simulink model "CanBusRagnarObserverPacketLoss"  (R2021b)
settings: Solver=VariableStepAuto  StartTime=0.0  StopTime=1.5  RelTol=1e-3
values from neighbouring files (symbols this model uses):
  F_mimo = -place(A,B,Desired_poles)    [SS_MIMO.m]
  L_mimo = -place(A',C',Desired_poles_obs)'    [SS_MIMO.m]
  sys_mimo = ss(A,B,C,0)    [SS_MIMO.m]
libraries: simulink_extras x8, truetime x6, dspsrcs4 x1
settings Model: Creator=mozzr  LastModifiedBy=mozzr
settings SolverCC: AlgebraicLoopSolver=TrustRegion

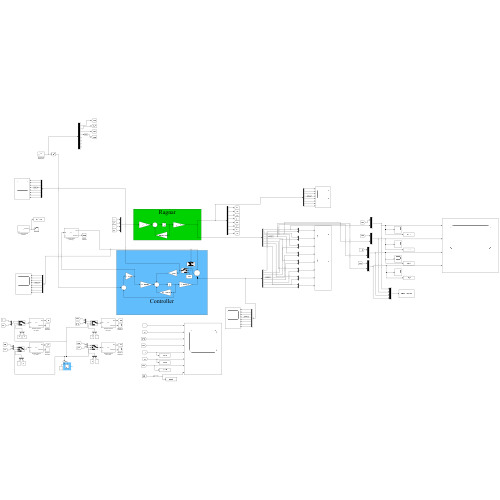
[thumbnail: Simulink's stored preview of the top-level diagram]
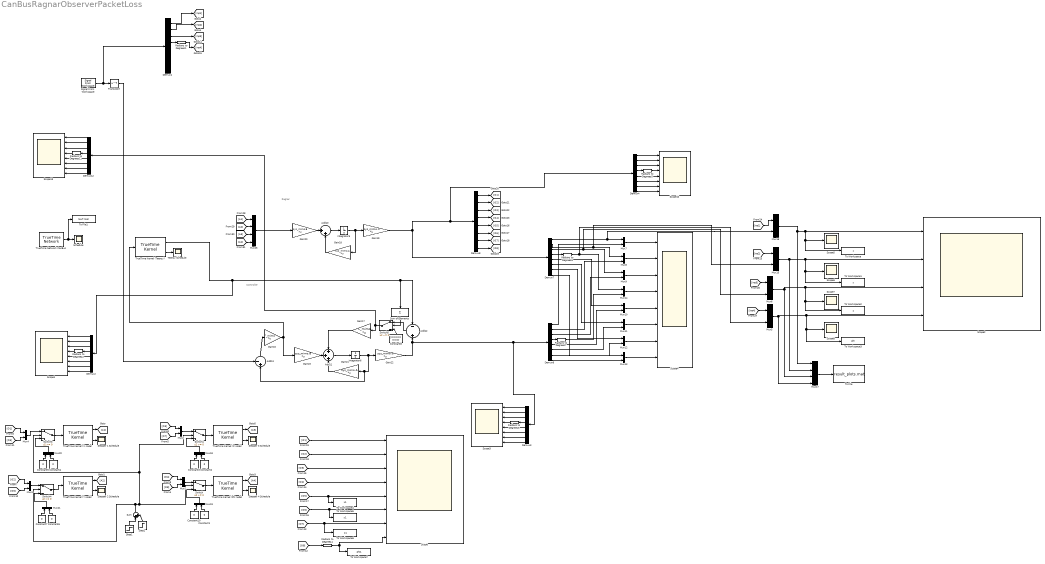
== system CanBusRagnarObserverPacketLoss ==
  note: Ragnar
  note: Controller
  Add10 : Sum  Inputs=|++
  Add11 : Sum  Inputs=+++
  Add12 : Sum  Inputs=-+
  Add13 : Sum  Inputs=-+|
  Constant{1..7,10} (8 alike) : Constant  Value=0
  Constant8 : Constant  Value=[0 0 0 0 0 0 0 0]'
  Demux{1..4,6..8,12} (8 alike) : Demux  Outputs=8
  Gain16 : Gain  Gain=F_mimo  Multiplication=Matrix(K*u)
  Gain17 : Gain  Gain=L_mimo  Multiplication=Matrix(K*u)
  Gain18 : Gain  Gain=sys_mimo.A  Multiplication=Matrix(K*u)
  Gain19 : Gain  Gain=sys_mimo.C  Multiplication=Matrix(K*u)
  Gain20 : Gain  Gain=sys_mimo.B  Multiplication=Matrix(K*u)
  Gain21 : Gain  Gain=sys_mimo.A  Multiplication=Matrix(K*u)
  Gain22 : Gain  Gain=sys_mimo.C  Multiplication=Matrix(K*u)
  Gain23 : Gain  Gain=sys_mimo.B  Multiplication=Matrix(K*u)
  Integrator5 : Integrator  InitialCondition=[0.01 0.51 -0.39 deg2rad(95) 0 0 0 0]'
  Integrator6 : Integrator  InitialCondition=[0.01 0.51 -0.39 deg2rad(95) 0 0 0 0]'
  Mux{1..16,18..21} (20 alike) : Mux  Inputs=2
  Mux17 : Mux
  Mux26 : Mux
  Radians to Degrees{1..7,11} (8 alike) : simulink_extras/Transformations/Radians to Degrees
  Schedule : Scope
  Scope{,1,3..4,10,13} (6 alike) : Scope  NumInputPorts=8
  Scope2 : Scope  NumInputPorts=4
  Scope{5..8} (4 alike) : Scope
  Signal From Workspace : dspsrcs4/Signal From Workspace  X=ref  Ts=0.5  nsamps=1  OutputAfterFinalValue=Holding final value  ignoreOrWarnInputAndFrameLengths=off  OutputFrames=off
  Step1 : Step  Time=0.7  Before=1  After=-1  SampleTime=0
  Step2 : Step  Time=0.9  After=2  SampleTime=0
  Stepper 1 Schedule : Scope
  Stepper 2 Schedule : Scope
  Stepper 3 Schedule : Scope
  Stepper 4 Schedule : Scope
  Sum : Sum  Inputs=|++
  Sum of Elements : Sum  Inputs=1
  Switch{,1,3..4} (4 alike) : Switch
  Switch5 : Switch  Criteria=u2 ~= 0  Threshold=1
  Teensy Schedule : Scope
  To File : ToFile  Filename=result_plots.mat  SaveFormat=Timeseries
  To File1 : ToFile  Filename=NwT.mat  SaveFormat=Timeseries
  To Workspace : ToWorkspace  VariableName=x  SaveFormat=Timeseries  SampleTime=-1
  To Workspace1 : ToWorkspace  VariableName=y  SaveFormat=Timeseries  SampleTime=-1
  To Workspace2 : ToWorkspace  VariableName=z  SaveFormat=Timeseries  SampleTime=-1
  To Workspace3 : ToWorkspace  VariableName=phi  SaveFormat=Timeseries  SampleTime=-1
  To Workspace4 : ToWorkspace  VariableName=x1  SaveFormat=Timeseries  SampleTime=-1
  To Workspace5 : ToWorkspace  VariableName=y1  SaveFormat=Timeseries  SampleTime=-1
  To Workspace6 : ToWorkspace  VariableName=z1  SaveFormat=Timeseries  SampleTime=-1
  To Workspace7 : ToWorkspace  VariableName=phi1  SaveFormat=Timeseries  SampleTime=-1
  Transpose : Math  Operator=transpose  SaturateOnIntegerOverflow=on
  TrueTime Kernel (Phi node) : truetime/TrueTime Kernel  sfun=nodePhi_init  args=[]  ninputsoutputs=[2 1]  ntriggers=0  trigtype=falling  nwnodenbr=[1 5]  clockoffsetdrift=[0 0]  schedoutput=on  battery=off  poweroutput=off  label=1: 5
  TrueTime Kernel (Teensy) : truetime/TrueTime Kernel  sfun=Teensy_init  args=[]  ninputsoutputs=[4 8]  ntriggers=0  trigtype=falling  nwnodenbr=[1 1]  clockoffsetdrift=[0 0]  schedoutput=on  battery=off  poweroutput=off  label=1: 1
  TrueTime Kernel (X node) : truetime/TrueTime Kernel  sfun=nodeX_init  args=[]  ninputsoutputs=[2 1]  ntriggers=0  trigtype=falling  nwnodenbr=[1 2]  clockoffsetdrift=[0 0]  schedoutput=on  battery=off  poweroutput=off  label=1: 2
  TrueTime Kernel (Y node) : truetime/TrueTime Kernel  sfun=nodeY_init  args=[]  ninputsoutputs=[2 1]  ntriggers=0  trigtype=falling  nwnodenbr=[1 3]  clockoffsetdrift=[0 0]  schedoutput=on  battery=off  poweroutput=off  label=1: 3
  TrueTime Kernel (Z node) : truetime/TrueTime Kernel  sfun=nodeZ_init  args=[]  ninputsoutputs=[2 1]  ntriggers=0  trigtype=falling  nwnodenbr=[1 4]  clockoffsetdrift=[0 0]  schedoutput=on  battery=off  poweroutput=off  label=1: 4
  TrueTime Network CanBus : truetime/TrueTime Network  nwtype=CSMA/AMP (CAN)  nwnbr=1  nnodes=5  rate=10000000  minsize=512  lossprob=0  seed=0  bandwidths=[0.5 0.5]  slotsize=512  schedule=[1 1 2]  memsize=80000  buftype=Common buffer  overflow=Retransmit  dynSchedule=0  miniSlotSize=0  NIT=0  QSortMode=FIFO  sync=0  irtSchedule=0  nrtLength=0  nodeGraph=0  scheduleoutput=on
  wires:
  TrueTime Kernel (Teensy)/2 -> Teensy Schedule/1
  TrueTime Network CanBus/1 -> To File1/1, Schedule/1
  [O7] -> To Workspace6/1, Scope/7
  [O4] -> Scope/4
  [O3] -> Scope/3
  [O5] -> To Workspace4/1, Scope/5
  [O6] -> To Workspace5/1, Scope/6
  [O2] -> Scope/2
  [O1] -> Scope/1
  Mux12/1 -> Scope4/7
  Mux7/1 -> Scope4/1
  Demux6/5 -> Mux10/2
  Mux11/1 -> Scope4/6
  Demux7/7 -> Mux12/1
  Demux6/1 -> Mux7/2
  Radians to Degrees7/1 -> Mux14/2
  Demux6/6 -> Mux11/2
  Demux6/7 -> Mux12/2
  Demux7/2 -> Mux15/2, Mux8/1
  Mux10/1 -> Scope4/5
  Demux6/2 -> Mux8/2
  Demux7/5 -> Mux10/1
  Mux13/1 -> Scope4/8
  Demux7/6 -> Mux11/1
  Radians to Degrees6/1 -> Mux5/2, Mux14/1
  Demux6/8 -> Mux13/2
  Demux7/8 -> Mux13/1
  Mux14/1 -> Scope4/4
  Demux6/4 -> Radians to Degrees7/1
  Demux6/3 -> Mux9/2
  Demux7/1 -> Mux16/2, Mux7/1
  Mux9/1 -> Scope4/3
  Demux7/4 -> Radians to Degrees6/1
  Demux7/3 -> Mux6/2, Mux9/1
  Mux8/1 -> Scope4/2
  Mux5/1 -> To Workspace3/1, Scope8/1, Scope2/4, Mux17/4
  Mux6/1 -> To Workspace2/1, Scope7/1, Scope2/3, Mux17/3
  Mux15/1 -> Mux17/2, To Workspace1/1, Scope6/1, Scope2/2
  Mux16/1 -> Mux17/1, To Workspace/1, Scope5/1, Scope2/1
  Demux1/4 -> Radians to Degrees1/1
  Demux1/1 -> [inp1]
  Demux1/2 -> [inp2]
  Demux1/3 -> [inp3]
  Radians to Degrees1/1 -> [inp4]
  [inp1] -> Mux16/1
  [inp2] -> Mux15/1
  [inp3] -> Mux6/1
  [inp4] -> Mux5/1
  Mux17/1 -> To File/1
  Gain21/1 -> Add11/3
  Add13/1 -> Gain16/1
  Gain23/1 -> Add11/2
  Gain16/1 -> TrueTime Kernel (Teensy)/1, Gain23/1
  Integrator5/1 -> Gain18/1, Gain19/1
  Gain18/1 -> Add10/2
  Gain20/1 -> Add10/1
  Add11/1 -> Integrator6/1
  Gain22/1 -> Demux3/1, Demux6/1, Add12/2
  Add10/1 -> Integrator5/1
  Gain17/1 -> Add11/1
  Integrator6/1 -> Add13/2, Gain21/1, Gain22/1
  Demux8/8 -> [O8]
  Demux8/7 -> [O7]
  Demux8/4 -> [O4]
  Demux8/5 -> [O5]
  Demux8/3 -> [O3]
  Demux8/1 -> [O1]
  Demux8/2 -> [O2]
  Demux8/6 -> [O6]
  [A4] -> Mux26/4
  [A3] -> Mux26/3
  [A2] -> Mux26/2
  [A1] -> Mux26/1
  Mux26/1 -> Gain20/1
  Signal From Workspace/1 -> Demux1/1, Transpose/1
  Transpose/1 -> Add13/1
  Demux4/6 -> Scope10/6
  Demux4/8 -> Scope10/8
  Demux4/2 -> Scope10/2
  Demux4/1 -> Scope10/1
  Demux4/7 -> Scope10/7
  Demux4/3 -> Scope10/3
  Demux4/4 -> Radians to Degrees5/1
  Demux4/5 -> Scope10/5
  Radians to Degrees5/1 -> Scope10/4
  Gain19/1 -> Demux4/1, Demux8/1, Demux7/1
  Demux12/6 -> Scope13/6
  Demux12/4 -> Radians to Degrees11/1
  Demux12/1 -> Scope13/1
  Demux12/8 -> Scope13/8
  Demux12/5 -> Scope13/5
  Radians to Degrees11/1 -> Scope13/4
  Demux12/2 -> Scope13/2
  Demux12/3 -> Scope13/3
  Demux12/7 -> Scope13/7
  [O2] -> Mux3/1
  Mux21/1 -> Switch4/3
  Constant7/1 -> Mux21/1
  [O1] -> Mux4/1
  Step1/1 -> Sum/1
  TrueTime Kernel (X node)/2 -> Stepper 1 Schedule/1
  Constant1/1 -> Mux19/2
  Constant5/1 -> Mux20/1
  Switch1/1 -> TrueTime Kernel (Z node)/1
  TrueTime Kernel (Phi node)/1 -> [A4]
  Mux20/1 -> Switch3/3
  Switch4/1 -> TrueTime Kernel (Y node)/1
  Constant4/1 -> Mux20/2
  Mux3/1 -> Switch4/1
  [O8] -> Mux1/2
  Mux4/1 -> Switch3/1
  Mux18/1 -> Switch1/3
  Constant2/1 -> Mux18/2
  Step2/1 -> Sum/2
  TrueTime Kernel (Y node)/2 -> Stepper 2 Schedule/1
  Sum/1 -> Switch3/2, Switch1/2, Switch/2, Switch4/2
  Switch/1 -> TrueTime Kernel (Phi node)/1
  Switch3/1 -> TrueTime Kernel (X node)/1
  Constant10/1 -> Mux19/1
  Mux19/1 -> Switch/3
  Mux1/1 -> Switch/1
  [O5] -> Mux4/2
  [O4] -> Mux1/1
  [O6] -> Mux3/2
  Mux2/1 -> Switch1/1
  [O7] -> Mux2/2
  TrueTime Kernel (Z node)/2 -> Stepper 3 Schedule/1
  Constant3/1 -> Mux18/1
  TrueTime Kernel (Z node)/1 -> [A3]
  TrueTime Kernel (X node)/1 -> [A1]
  TrueTime Kernel (Phi node)/2 -> Stepper 4 Schedule/1
  [O3] -> Mux2/1
  TrueTime Kernel (Y node)/1 -> [A2]
  Constant6/1 -> Mux21/2
  Sum of Elements/1 -> Switch5/2
  Add12/1 -> Switch5/1
  Constant8/1 -> Switch5/3
  Switch5/1 -> Demux12/1, Gain17/1
  Demux2/7 -> Scope1/7
  Demux2/8 -> Scope1/8
  Radians to Degrees2/1 -> Scope1/4
  Demux2/1 -> Scope1/1
  Demux2/5 -> Scope1/5
  Demux2/6 -> Scope1/6
  Demux2/3 -> Scope1/3
  Demux2/4 -> Radians to Degrees2/1
  Demux2/2 -> Scope1/2
  Demux3/7 -> Scope3/7
  Demux3/8 -> Scope3/8
  Radians to Degrees3/1 -> Scope3/4
  Demux3/1 -> Scope3/1
  Demux3/5 -> Scope3/5
  Demux3/6 -> Scope3/6
  Demux3/3 -> Scope3/3
  Demux3/4 -> Radians to Degrees3/1
  Demux3/2 -> Scope3/2
  TrueTime Kernel (Teensy)/1 -> Demux2/1, Sum of Elements/1, Add12/1
  [O8] -> Radians to Degrees4/1
  Radians to Degrees4/1 -> Scope/8, To Workspace7/1
